simulink model "two_parallel_full_model_simscape"  (R2023b)
settings: Solver=ode1be  StartTime=0.0  StopTime=simlength  FixedStep=ts_sim  MaxStep=ts_sim
undefined symbols (not defined in the file): fclock, fPWM_INV, fPWM_ZVS, gate_nominal_voltage, I_FS, Iout_dc_nom, ki_i_inv, ki_i_zvs, ki_v_inv, ki_v_zvs, kp_i_inv, kp_i_zvs, kp_v_inv, kp_v_zvs, LFi_dc, LFu_ac, magnitude, n10, omega_grid, RCFu_dc, RLFi_dc, RLFu_ac, tc, Tc, tPWM_ZVS, ts_afe, ts_inv, ts_zvs, ugrid_factor, Ugrid_phase_normalization_factor, un_eta_pu, un_xi_pu, up_xi_pu, v1_trafo, v2_trafo, V_FS, Vout_dc_nom
libraries: fl_lib x142, nesl_utility x55, single_phase_transformer_lib x4
(part 4 of 4)

== system two_parallel_full_model_simscape/zvs_modA/dc//dc with galvanic isolation/stage-1/h-bridge ==
  gate_commands : Inport
  Bus Selector : BusSelector  OutputSignals=gate_Q1,gate_Q2,gate_Q3,gate_Q4
  Current Sensor1 : fl_lib/Electrical/Electrical Sensors/Current Sensor
  Simulink-PS Converter{,1..3} (4 alike) : nesl_utility/Simulink-PS Converter  PhysicalDomain=network_engine_domain  SubClassName=ps_input  LeftPortType=input  RightPortType=output  PseudoPeriodic=off  Frequencies=[]  NoiseDistribution=none  NoiseParameters=[]  Unit=1  AffineConversion=on  FilteringAndDerivatives=provide  SimscapeFilterOrder=1  InputFilterTimeConstant=0.001  UdotUserProvided=0
  ileg_dc_inv : nesl_utility/PS-Simulink Converter  PhysicalDomain=network_engine_domain  SubClassName=ps_output  LeftPortType=input  RightPortType=output  PseudoPeriodic=off  Frequencies=[]  VectorFormat=1-D array  Unit=A  AffineConversion=on
  switch_1 : Subsystem
      settings: PortSchema="{\"entries\":[{\"content\":{\"sides\":[{\"content\":{\"connectorIds\":[\"LConn1\"]},\"type\":\"ConnectorPlacement.EquallySpacedRectSide\",\"uuid\":\"9277da8d-d460-43e6-8478-dd662f15d226\"},{\"content\":{\"connectorIds\":[],\"side\":\"RIGHT\"},\"type\":\"ConnectorPlacement.EquallySpacedRectSide\",\"uuid\":\"a7ece396-f1d9-4f4f-a05b-db1fc65d6e1d\"},{\"content\":{\"connectorIds\":[\"LConn2\"],\"side\":\"TOP\"},\"type\":\"ConnectorPlacement.EquallySpacedRectSide\",\"uuid\":\"fdd70777-e9cf-4317-afb6-cae87f75d5b0\"},{\"content\":{\"connectorIds\":[\"RConn1\"],\"side\":\"BOTTOM\"},\"type\":\"ConnectorPlacement.EquallySpacedRectSide\",\"uuid\":\"2353ed68-b1a1-4775-9ca9-31e268d5443b\"}]},\"type\":\"ConnectorPlacement.EquallySpacedConnector\",\"uuid\":\"d5479f4c-4e65-4791-adcb-73df11f88590\"}],\"packageUris\":[\"http://schema.mathworks.com/mf0/Connector/R2020b\"],\"version\":\"1.0\"}"
  switch_2 : Subsystem
      settings: PortSchema="{\"entries\":[{\"content\":{\"sides\":[{\"content\":{\"connectorIds\":[\"LConn1\"]},\"type\":\"ConnectorPlacement.EquallySpacedRectSide\",\"uuid\":\"9277da8d-d460-43e6-8478-dd662f15d226\"},{\"content\":{\"connectorIds\":[],\"side\":\"RIGHT\"},\"type\":\"ConnectorPlacement.EquallySpacedRectSide\",\"uuid\":\"a7ece396-f1d9-4f4f-a05b-db1fc65d6e1d\"},{\"content\":{\"connectorIds\":[\"LConn2\"],\"side\":\"TOP\"},\"type\":\"ConnectorPlacement.EquallySpacedRectSide\",\"uuid\":\"fdd70777-e9cf-4317-afb6-cae87f75d5b0\"},{\"content\":{\"connectorIds\":[\"RConn1\"],\"side\":\"BOTTOM\"},\"type\":\"ConnectorPlacement.EquallySpacedRectSide\",\"uuid\":\"2353ed68-b1a1-4775-9ca9-31e268d5443b\"}]},\"type\":\"ConnectorPlacement.EquallySpacedConnector\",\"uuid\":\"d5479f4c-4e65-4791-adcb-73df11f88590\"}],\"packageUris\":[\"http://schema.mathworks.com/mf0/Connector/R2020b\"],\"version\":\"1.0\"}"
  switch_3 : Subsystem
      settings: PortSchema="{\"entries\":[{\"content\":{\"sides\":[{\"content\":{\"connectorIds\":[\"LConn1\"]},\"type\":\"ConnectorPlacement.EquallySpacedRectSide\",\"uuid\":\"9277da8d-d460-43e6-8478-dd662f15d226\"},{\"content\":{\"connectorIds\":[],\"side\":\"RIGHT\"},\"type\":\"ConnectorPlacement.EquallySpacedRectSide\",\"uuid\":\"a7ece396-f1d9-4f4f-a05b-db1fc65d6e1d\"},{\"content\":{\"connectorIds\":[\"LConn2\"],\"side\":\"TOP\"},\"type\":\"ConnectorPlacement.EquallySpacedRectSide\",\"uuid\":\"fdd70777-e9cf-4317-afb6-cae87f75d5b0\"},{\"content\":{\"connectorIds\":[\"RConn1\"],\"side\":\"BOTTOM\"},\"type\":\"ConnectorPlacement.EquallySpacedRectSide\",\"uuid\":\"2353ed68-b1a1-4775-9ca9-31e268d5443b\"}]},\"type\":\"ConnectorPlacement.EquallySpacedConnector\",\"uuid\":\"d5479f4c-4e65-4791-adcb-73df11f88590\"}],\"packageUris\":[\"http://schema.mathworks.com/mf0/Connector/R2020b\"],\"version\":\"1.0\"}"
  switch_4 : Subsystem
      settings: PortSchema="{\"entries\":[{\"content\":{\"sides\":[{\"content\":{\"connectorIds\":[\"LConn1\"]},\"type\":\"ConnectorPlacement.EquallySpacedRectSide\",\"uuid\":\"9277da8d-d460-43e6-8478-dd662f15d226\"},{\"content\":{\"connectorIds\":[],\"side\":\"RIGHT\"},\"type\":\"ConnectorPlacement.EquallySpacedRectSide\",\"uuid\":\"a7ece396-f1d9-4f4f-a05b-db1fc65d6e1d\"},{\"content\":{\"connectorIds\":[\"LConn2\"],\"side\":\"TOP\"},\"type\":\"ConnectorPlacement.EquallySpacedRectSide\",\"uuid\":\"fdd70777-e9cf-4317-afb6-cae87f75d5b0\"},{\"content\":{\"connectorIds\":[\"RConn1\"],\"side\":\"BOTTOM\"},\"type\":\"ConnectorPlacement.EquallySpacedRectSide\",\"uuid\":\"2353ed68-b1a1-4775-9ca9-31e268d5443b\"}]},\"type\":\"ConnectorPlacement.EquallySpacedConnector\",\"uuid\":\"d5479f4c-4e65-4791-adcb-73df11f88590\"}],\"packageUris\":[\"http://schema.mathworks.com/mf0/Connector/R2020b\"],\"version\":\"1.0\"}"
  uac_1(+) : PMIOPort  Side=Left
  uac_1(-) : PMIOPort  Port=2  Side=Left
  udc(+) : PMIOPort  Port=3  Side=Right
  udc(-) : PMIOPort  Port=4  Side=Right
  tag scope: ileg_dc_inv=global
  wires:
  [gate_Q1] -> Simulink-PS Converter/1
  [gate_Q2] -> Simulink-PS Converter1/1
  [gate_Q3] -> Simulink-PS Converter2/1
  [gate_Q4] -> Simulink-PS Converter3/1
  gate_commands/1 -> Bus Selector/1
  ileg_dc_inv/1 -> [ileg_dc_inv]
  Bus Selector/1 -> [gate_Q1]  "<gate_Q1>"
  Bus Selector/2 -> [gate_Q2]  "<gate_Q2>"
  Bus Selector/3 -> [gate_Q3]  "<gate_Q3>"
  Bus Selector/4 -> [gate_Q4]  "<gate_Q4>"
  connections:
  Current Sensor1/LConn1 -- switch_3/LConn2 -- udc(+)/RConn1
  udc(-)/RConn1 -- switch_4/RConn1 -- switch_2/RConn1
  Simulink-PS Converter/RConn1 -- switch_1/LConn1
  switch_2/LConn1 -- Simulink-PS Converter1/RConn1
  switch_3/LConn1 -- Simulink-PS Converter2/RConn1
  switch_4/LConn1 -- Simulink-PS Converter3/RConn1
  uac_1(+)/RConn1 -- switch_2/LConn2 -- switch_1/RConn1
  uac_1(-)/RConn1 -- switch_4/LConn2 -- switch_3/RConn1
  Current Sensor1/RConn2 -- switch_1/LConn2
  Current Sensor1/RConn1 -- ileg_dc_inv/LConn1

== system two_parallel_full_model_simscape/zvs_modA/dc//dc with galvanic isolation/stage-2/two-phase-rectifier_tr1 ==
  Diode{,1,3..4} (4 alike) : fl_lib/Electrical/Electrical Elements/Diode  Vf=Vdon_diode V  Ron=Rdon_diode Ohm  Goff=1e-8 1/Ohm  i_specify=off  i_priority=None  i=0 A  i_nominal_specify=off  i_nominal_unit=A  i_nominal_value=1  v_specify=off  v_priority=None  v=0 V  v_nominal_specify=off  v_nominal_unit=V  v_nominal_value=1
  udc(+) : PMIOPort  Side=Right
  uac(+) : PMIOPort  Port=2  Side=Left
  uac(-) : PMIOPort  Port=3  Side=Left
  udc(-) : PMIOPort  Port=4  Side=Right
  connections:
  Diode/LConn1 -- Diode3/RConn1 -- uac(+)/RConn1
  Diode/RConn1 -- udc(+)/RConn1 -- Diode1/RConn1
  Diode3/LConn1 -- udc(-)/RConn1 -- Diode4/LConn1
  Diode4/RConn1 -- Diode1/LConn1 -- uac(-)/RConn1

== system two_parallel_full_model_simscape/zvs_modA/dc//dc with galvanic isolation/stage-2/two-phase-rectifier_tr2 ==
  Diode{,1,3..4} (4 alike) : fl_lib/Electrical/Electrical Elements/Diode  Vf=Vdon_diode V  Ron=Rdon_diode Ohm  Goff=1e-8 1/Ohm  i_specify=off  i_priority=None  i=0 A  i_nominal_specify=off  i_nominal_unit=A  i_nominal_value=1  v_specify=off  v_priority=None  v=0 V  v_nominal_specify=off  v_nominal_unit=V  v_nominal_value=1
  udc(+) : PMIOPort  Side=Right
  uac(+) : PMIOPort  Port=2  Side=Left
  uac(-) : PMIOPort  Port=3  Side=Left
  udc(-) : PMIOPort  Port=4  Side=Right
  connections:
  uac(-)/RConn1 -- Diode4/RConn1 -- Diode1/LConn1
  udc(-)/RConn1 -- Diode4/LConn1 -- Diode3/LConn1
  udc(+)/RConn1 -- Diode1/RConn1 -- Diode/RConn1
  uac(+)/RConn1 -- Diode3/RConn1 -- Diode/LConn1

== system two_parallel_full_model_simscape/zvs_modA/zvs_ctrl/references/voltage_reference ==
  Constant1 : Constant  Value=Vout_dc_nom
  Manual Switch : ManualSwitch
  Rate Limiter : RateLimiter  RisingSlewLimit=Vout_dc_nom  FallingSlewLimit=-Vout_dc_nom  SampleTimeMode=inherited
  Step : Step  Time=0.25  After=20  SampleTime=0
  Step1 : Step  Time=0.45  After=480  SampleTime=0
  Step2 : Step  Time=0.75  After=480  SampleTime=0
  Step3 : Step  After=780  SampleTime=0
  Sum : Sum  Inputs=|++
  Sum1 : Sum  Inputs=|+-
  Sum2 : Sum  Inputs=|++
  To Workspace2 : ToWorkspace  VariableName=vout_ref_modA_sim  SampleTime=ts_zvs
      settings: MaxDataPoints=Ns_zvs
  Vout_dc_nom : Step  Time=1e-3  After=Vout_dc_nom  SampleTime=0
  vout_ref : Outport
  wires:
  Step/1 -> Sum/1
  Step1/1 -> Sum/2
  Sum/1 -> Sum1/1
  Step2/1 -> Sum1/2
  Sum1/1 -> Sum2/1
  Step3/1 -> Sum2/2
  Sum2/1 -> Manual Switch/2
  Vout_dc_nom/1 -> Rate Limiter/1
  Manual Switch/1 -> To Workspace2/1, vout_ref/1
  Rate Limiter/1 -> Manual Switch/1

== system two_parallel_full_model_simscape/zvs_modA/zvs_ctrl/vi ctrl/Iout Ctrl ==
  iout_ref : Inport
  iout : Inport  Port=2
  Product : Product
  Rate Limiter : RateLimiter  FallingSlewLimit=0  SampleTimeMode=inherited
  Saturation1 : Saturate  UpperLimit=1  LowerLimit=0  OutDataTypeStr=double
  Step : Step  Time=0.1  SampleTime=0
  Sum2 : Sum  Inputs=+-  OutDataTypeStr=double  AccumDataTypeStr=double  SaturateOnIntegerOverflow=on
  To Workspace2 : ToWorkspace  VariableName=iout_ref_dsp_modA_sim  SampleTime=ts_zvs
      settings: MaxDataPoints=Ns_zvs
  To Workspace9 : ToWorkspace  VariableName=iout_dsp_modA_sim  SampleTime=ts_zvs
      settings: MaxDataPoints=Ns_zvs
  iout_ctrl : Subsystem
  ctrli_out : Outport
  wires:
  iout_ctrl/1(ctrli_out) -> ctrli_out/1
  iout/1 -> To Workspace9/1, Sum2/2
  iout_ref/1 -> Sum2/1, To Workspace2/1
  Rate Limiter/1 -> Saturation1/1
  Saturation1/1 -> Product/1
  Step/1 -> Rate Limiter/1
  Sum2/1 -> Product/2
  Product/1 -> iout_ctrl/1(i_tilde)

== system two_parallel_full_model_simscape/zvs_modA/zvs_ctrl/vi ctrl/Vout Ctrl ==
  vout_ref : Inport
  vout : Inport  Port=2
  Product : Product
  Rate Limiter : RateLimiter  FallingSlewLimit=0  SampleTimeMode=inherited
  Saturation1 : Saturate  UpperLimit=1  LowerLimit=0  OutDataTypeStr=double
  Step : Step  Time=0.1  SampleTime=0
  Sum2 : Sum  Inputs=+-  OutDataTypeStr=double  AccumDataTypeStr=double  SaturateOnIntegerOverflow=on
  To Workspace2 : ToWorkspace  VariableName=vout_ref_dsp_modA_sim  SampleTime=ts_zvs
      settings: MaxDataPoints=Ns_zvs
  To Workspace9 : ToWorkspace  VariableName=vout_dsp_modA_sim  SampleTime=ts_zvs
      settings: MaxDataPoints=Ns_zvs
  vout_ctrl : Subsystem
  ctrlv_out : Outport
  wires:
  vout_ref/1 -> To Workspace2/1, Sum2/1
  vout/1 -> To Workspace9/1, Sum2/2
  vout_ctrl/1(ctrlv_out) -> ctrlv_out/1
  Sum2/1 -> Product/2
  Product/1 -> vout_ctrl/1(ixi_tilde)
  Step/1 -> Rate Limiter/1
  Rate Limiter/1 -> Saturation1/1
  Saturation1/1 -> Product/1

== system two_parallel_full_model_simscape/zvs_modB/dc//dc with galvanic isolation/stage-1/h-bridge ==
  gate_commands : Inport
  Bus Selector : BusSelector  OutputSignals=gate_Q1,gate_Q2,gate_Q3,gate_Q4
  Simulink-PS Converter{,1..3} (4 alike) : nesl_utility/Simulink-PS Converter  PhysicalDomain=network_engine_domain  SubClassName=ps_input  LeftPortType=input  RightPortType=output  PseudoPeriodic=off  Frequencies=[]  NoiseDistribution=none  NoiseParameters=[]  Unit=1  AffineConversion=on  FilteringAndDerivatives=provide  SimscapeFilterOrder=1  InputFilterTimeConstant=0.001  UdotUserProvided=0
  switch_1 : Subsystem
      settings: PortSchema="{\"entries\":[{\"content\":{\"sides\":[{\"content\":{\"connectorIds\":[\"LConn1\"]},\"type\":\"ConnectorPlacement.EquallySpacedRectSide\",\"uuid\":\"9277da8d-d460-43e6-8478-dd662f15d226\"},{\"content\":{\"connectorIds\":[],\"side\":\"RIGHT\"},\"type\":\"ConnectorPlacement.EquallySpacedRectSide\",\"uuid\":\"a7ece396-f1d9-4f4f-a05b-db1fc65d6e1d\"},{\"content\":{\"connectorIds\":[\"LConn2\"],\"side\":\"TOP\"},\"type\":\"ConnectorPlacement.EquallySpacedRectSide\",\"uuid\":\"fdd70777-e9cf-4317-afb6-cae87f75d5b0\"},{\"content\":{\"connectorIds\":[\"RConn1\"],\"side\":\"BOTTOM\"},\"type\":\"ConnectorPlacement.EquallySpacedRectSide\",\"uuid\":\"2353ed68-b1a1-4775-9ca9-31e268d5443b\"}]},\"type\":\"ConnectorPlacement.EquallySpacedConnector\",\"uuid\":\"d5479f4c-4e65-4791-adcb-73df11f88590\"}],\"packageUris\":[\"http://schema.mathworks.com/mf0/Connector/R2020b\"],\"version\":\"1.0\"}"
  switch_2 : Subsystem
      settings: PortSchema="{\"entries\":[{\"content\":{\"sides\":[{\"content\":{\"connectorIds\":[\"LConn1\"]},\"type\":\"ConnectorPlacement.EquallySpacedRectSide\",\"uuid\":\"9277da8d-d460-43e6-8478-dd662f15d226\"},{\"content\":{\"connectorIds\":[],\"side\":\"RIGHT\"},\"type\":\"ConnectorPlacement.EquallySpacedRectSide\",\"uuid\":\"a7ece396-f1d9-4f4f-a05b-db1fc65d6e1d\"},{\"content\":{\"connectorIds\":[\"LConn2\"],\"side\":\"TOP\"},\"type\":\"ConnectorPlacement.EquallySpacedRectSide\",\"uuid\":\"fdd70777-e9cf-4317-afb6-cae87f75d5b0\"},{\"content\":{\"connectorIds\":[\"RConn1\"],\"side\":\"BOTTOM\"},\"type\":\"ConnectorPlacement.EquallySpacedRectSide\",\"uuid\":\"2353ed68-b1a1-4775-9ca9-31e268d5443b\"}]},\"type\":\"ConnectorPlacement.EquallySpacedConnector\",\"uuid\":\"d5479f4c-4e65-4791-adcb-73df11f88590\"}],\"packageUris\":[\"http://schema.mathworks.com/mf0/Connector/R2020b\"],\"version\":\"1.0\"}"
  switch_3 : Subsystem
      settings: PortSchema="{\"entries\":[{\"content\":{\"sides\":[{\"content\":{\"connectorIds\":[\"LConn1\"]},\"type\":\"ConnectorPlacement.EquallySpacedRectSide\",\"uuid\":\"9277da8d-d460-43e6-8478-dd662f15d226\"},{\"content\":{\"connectorIds\":[],\"side\":\"RIGHT\"},\"type\":\"ConnectorPlacement.EquallySpacedRectSide\",\"uuid\":\"a7ece396-f1d9-4f4f-a05b-db1fc65d6e1d\"},{\"content\":{\"connectorIds\":[\"LConn2\"],\"side\":\"TOP\"},\"type\":\"ConnectorPlacement.EquallySpacedRectSide\",\"uuid\":\"fdd70777-e9cf-4317-afb6-cae87f75d5b0\"},{\"content\":{\"connectorIds\":[\"RConn1\"],\"side\":\"BOTTOM\"},\"type\":\"ConnectorPlacement.EquallySpacedRectSide\",\"uuid\":\"2353ed68-b1a1-4775-9ca9-31e268d5443b\"}]},\"type\":\"ConnectorPlacement.EquallySpacedConnector\",\"uuid\":\"d5479f4c-4e65-4791-adcb-73df11f88590\"}],\"packageUris\":[\"http://schema.mathworks.com/mf0/Connector/R2020b\"],\"version\":\"1.0\"}"
  switch_4 : Subsystem
      settings: PortSchema="{\"entries\":[{\"content\":{\"sides\":[{\"content\":{\"connectorIds\":[\"LConn1\"]},\"type\":\"ConnectorPlacement.EquallySpacedRectSide\",\"uuid\":\"9277da8d-d460-43e6-8478-dd662f15d226\"},{\"content\":{\"connectorIds\":[],\"side\":\"RIGHT\"},\"type\":\"ConnectorPlacement.EquallySpacedRectSide\",\"uuid\":\"a7ece396-f1d9-4f4f-a05b-db1fc65d6e1d\"},{\"content\":{\"connectorIds\":[\"LConn2\"],\"side\":\"TOP\"},\"type\":\"ConnectorPlacement.EquallySpacedRectSide\",\"uuid\":\"fdd70777-e9cf-4317-afb6-cae87f75d5b0\"},{\"content\":{\"connectorIds\":[\"RConn1\"],\"side\":\"BOTTOM\"},\"type\":\"ConnectorPlacement.EquallySpacedRectSide\",\"uuid\":\"2353ed68-b1a1-4775-9ca9-31e268d5443b\"}]},\"type\":\"ConnectorPlacement.EquallySpacedConnector\",\"uuid\":\"d5479f4c-4e65-4791-adcb-73df11f88590\"}],\"packageUris\":[\"http://schema.mathworks.com/mf0/Connector/R2020b\"],\"version\":\"1.0\"}"
  uac_1(+) : PMIOPort  Side=Left
  uac_1(-) : PMIOPort  Port=2  Side=Left
  udc(+) : PMIOPort  Port=3  Side=Right
  udc(-) : PMIOPort  Port=4  Side=Right
  wires:
  Bus Selector/4 -> [gate_Q4]  "<gate_Q4>"
  Bus Selector/3 -> [gate_Q3]  "<gate_Q3>"
  Bus Selector/2 -> [gate_Q2]  "<gate_Q2>"
  Bus Selector/1 -> [gate_Q1]  "<gate_Q1>"
  gate_commands/1 -> Bus Selector/1
  [gate_Q4] -> Simulink-PS Converter3/1
  [gate_Q3] -> Simulink-PS Converter2/1
  [gate_Q2] -> Simulink-PS Converter1/1
  [gate_Q1] -> Simulink-PS Converter/1
  connections:
  switch_3/RConn1 -- switch_4/LConn2 -- uac_1(-)/RConn1
  switch_1/RConn1 -- switch_2/LConn2 -- uac_1(+)/RConn1
  switch_4/LConn1 -- Simulink-PS Converter3/RConn1
  switch_3/LConn1 -- Simulink-PS Converter2/RConn1
  switch_2/LConn1 -- Simulink-PS Converter1/RConn1
  Simulink-PS Converter/RConn1 -- switch_1/LConn1
  switch_2/RConn1 -- switch_4/RConn1 -- udc(-)/RConn1
  udc(+)/RConn1 -- switch_3/LConn2 -- switch_1/LConn2

== system two_parallel_full_model_simscape/zvs_modB/dc//dc with galvanic isolation/stage-2/two-phase-rectifier_tr1 ==
  Diode{,1,3..4} (4 alike) : fl_lib/Electrical/Electrical Elements/Diode  Vf=Vdon_diode V  Ron=Rdon_diode Ohm  Goff=1e-8 1/Ohm  i_specify=off  i_priority=None  i=0 A  i_nominal_specify=off  i_nominal_unit=A  i_nominal_value=1  v_specify=off  v_priority=None  v=0 V  v_nominal_specify=off  v_nominal_unit=V  v_nominal_value=1
  udc(+) : PMIOPort  Side=Right
  uac(+) : PMIOPort  Port=2  Side=Left
  uac(-) : PMIOPort  Port=3  Side=Left
  udc(-) : PMIOPort  Port=4  Side=Right
  connections:
  uac(-)/RConn1 -- Diode1/LConn1 -- Diode4/RConn1
  Diode4/LConn1 -- udc(-)/RConn1 -- Diode3/LConn1
  Diode1/RConn1 -- udc(+)/RConn1 -- Diode/RConn1
  uac(+)/RConn1 -- Diode3/RConn1 -- Diode/LConn1

== system two_parallel_full_model_simscape/zvs_modB/dc//dc with galvanic isolation/stage-2/two-phase-rectifier_tr2 ==
  Diode{,1,3..4} (4 alike) : fl_lib/Electrical/Electrical Elements/Diode  Vf=Vdon_diode V  Ron=Rdon_diode Ohm  Goff=1e-8 1/Ohm  i_specify=off  i_priority=None  i=0 A  i_nominal_specify=off  i_nominal_unit=A  i_nominal_value=1  v_specify=off  v_priority=None  v=0 V  v_nominal_specify=off  v_nominal_unit=V  v_nominal_value=1
  udc(+) : PMIOPort  Side=Right
  uac(+) : PMIOPort  Port=2  Side=Left
  uac(-) : PMIOPort  Port=3  Side=Left
  udc(-) : PMIOPort  Port=4  Side=Right
  connections:
  Diode/LConn1 -- Diode3/RConn1 -- uac(+)/RConn1
  Diode/RConn1 -- Diode1/RConn1 -- udc(+)/RConn1
  Diode3/LConn1 -- Diode4/LConn1 -- udc(-)/RConn1
  Diode1/LConn1 -- Diode4/RConn1 -- uac(-)/RConn1

== system two_parallel_full_model_simscape/zvs_modB/zvs_ctrl/references/voltage_reference ==
  Constant1 : Constant  Value=Vout_dc_nom
  Manual Switch : ManualSwitch
  Rate Limiter : RateLimiter  RisingSlewLimit=Vout_dc_nom  FallingSlewLimit=-Vout_dc_nom  SampleTimeMode=inherited
  Step : Step  Time=0.25  After=20  SampleTime=0
  Step1 : Step  Time=0.45  After=480  SampleTime=0
  Step2 : Step  Time=0.75  After=480  SampleTime=0
  Step3 : Step  After=780  SampleTime=0
  Sum : Sum  Inputs=|++
  Sum1 : Sum  Inputs=|+-
  Sum2 : Sum  Inputs=|++
  Vout_dc_nom : Step  Time=1e-3  After=Vout_dc_nom  SampleTime=0
  vout_ref : Outport
  wires:
  Rate Limiter/1 -> Manual Switch/1
  Manual Switch/1 -> vout_ref/1
  Vout_dc_nom/1 -> Rate Limiter/1
  Sum2/1 -> Manual Switch/2
  Step3/1 -> Sum2/2
  Sum1/1 -> Sum2/1
  Step2/1 -> Sum1/2
  Sum/1 -> Sum1/1
  Step1/1 -> Sum/2
  Step/1 -> Sum/1

== system two_parallel_full_model_simscape/zvs_modB/zvs_ctrl/vi ctrl/Iout Ctrl ==
  iout_ref : Inport
  iout : Inport  Port=2
  Product : Product
  Rate Limiter : RateLimiter  FallingSlewLimit=0  SampleTimeMode=inherited
  Saturation1 : Saturate  UpperLimit=1  LowerLimit=0  OutDataTypeStr=double
  Step : Step  Time=0.1  SampleTime=0
  Sum2 : Sum  Inputs=+-  OutDataTypeStr=double  AccumDataTypeStr=double  SaturateOnIntegerOverflow=on
  To Workspace2 : ToWorkspace  VariableName=iout_ref_dsp_modB_sim  SampleTime=ts_zvs
      settings: MaxDataPoints=Ns_zvs
  To Workspace9 : ToWorkspace  VariableName=iout_dsp_modB_sim  SampleTime=ts_zvs
      settings: MaxDataPoints=Ns_zvs
  iout_ctrl : Subsystem
  ctrli_out : Outport
  wires:
  Product/1 -> iout_ctrl/1(i_tilde)
  Sum2/1 -> Product/2
  Step/1 -> Rate Limiter/1
  Saturation1/1 -> Product/1
  Rate Limiter/1 -> Saturation1/1
  iout_ref/1 -> To Workspace2/1, Sum2/1
  iout/1 -> Sum2/2, To Workspace9/1
  iout_ctrl/1(ctrli_out) -> ctrli_out/1

== system two_parallel_full_model_simscape/zvs_modB/zvs_ctrl/vi ctrl/Vout Ctrl ==
  vout_ref : Inport
  vout : Inport  Port=2
  Product : Product
  Rate Limiter : RateLimiter  FallingSlewLimit=0  SampleTimeMode=inherited
  Saturation1 : Saturate  UpperLimit=1  LowerLimit=0  OutDataTypeStr=double
  Step : Step  Time=0.1  SampleTime=0
  Sum2 : Sum  Inputs=+-  OutDataTypeStr=double  AccumDataTypeStr=double  SaturateOnIntegerOverflow=on
  To Workspace2 : ToWorkspace  VariableName=vout_ref_dsp_modB_sim  SampleTime=ts_zvs
      settings: MaxDataPoints=Ns_zvs
  To Workspace9 : ToWorkspace  VariableName=vout_dsp_modB_sim  SampleTime=ts_zvs
      settings: MaxDataPoints=Ns_zvs
  vout_ctrl : Subsystem
  ctrlv_out : Outport
  wires:
  Saturation1/1 -> Product/1
  Rate Limiter/1 -> Saturation1/1
  Step/1 -> Rate Limiter/1
  Product/1 -> vout_ctrl/1(ixi_tilde)
  Sum2/1 -> Product/2
  vout_ctrl/1(ctrlv_out) -> ctrlv_out/1
  vout/1 -> Sum2/2, To Workspace9/1
  vout_ref/1 -> Sum2/1, To Workspace2/1

== system two_parallel_full_model_simscape/zvs_modA/dc//dc with galvanic isolation/stage-1/h-bridge/switch_1 ==
  Diode : fl_lib/Electrical/Electrical Elements/Diode  Vf=Vdon_diode V  Ron=Rdon_diode Ohm  Goff=1e-8 1/Ohm  i_specify=off  i_priority=None  i=0 A  i_nominal_specify=off  i_nominal_unit=A  i_nominal_value=1  v_specify=off  v_priority=None  v=0 V  v_nominal_specify=off  v_nominal_unit=V  v_nominal_value=1
  Switch : fl_lib/Electrical/Electrical Elements/Switch  R_closed=Ron Ohm  G_open=1e-8 1/Ohm  Threshold=7.5  i_specify=off  i_priority=None  i=0 A  i_nominal_specify=off  i_nominal_unit=A  i_nominal_value=1  v_specify=off  v_priority=None  v=0 V  v_nominal_specify=off  v_nominal_unit=V  v_nominal_value=1
  G : PMIOPort  Side=Left
  C : PMIOPort  Port=2  Side=Left
  E : PMIOPort  Port=3  Side=Right
  connections:
  Switch/RConn2 -- C/RConn1 -- Diode/RConn1
  Switch/RConn1 -- G/RConn1
  Switch/LConn1 -- E/RConn1 -- Diode/LConn1

== system two_parallel_full_model_simscape/zvs_modA/dc//dc with galvanic isolation/stage-1/h-bridge/switch_2 ==
  Diode : fl_lib/Electrical/Electrical Elements/Diode  Vf=Vdon_diode V  Ron=Rdon_diode Ohm  Goff=1e-8 1/Ohm  i_specify=off  i_priority=None  i=0 A  i_nominal_specify=off  i_nominal_unit=A  i_nominal_value=1  v_specify=off  v_priority=None  v=0 V  v_nominal_specify=off  v_nominal_unit=V  v_nominal_value=1
  Switch : fl_lib/Electrical/Electrical Elements/Switch  R_closed=Ron Ohm  G_open=1e-8 1/Ohm  Threshold=7.5  i_specify=off  i_priority=None  i=0 A  i_nominal_specify=off  i_nominal_unit=A  i_nominal_value=1  v_specify=off  v_priority=None  v=0 V  v_nominal_specify=off  v_nominal_unit=V  v_nominal_value=1
  G : PMIOPort  Side=Left
  C : PMIOPort  Port=2  Side=Left
  E : PMIOPort  Port=3  Side=Right
  connections:
  Diode/LConn1 -- E/RConn1 -- Switch/LConn1
  Switch/RConn1 -- G/RConn1
  Diode/RConn1 -- C/RConn1 -- Switch/RConn2

== system two_parallel_full_model_simscape/zvs_modA/dc//dc with galvanic isolation/stage-1/h-bridge/switch_3 ==
  Diode : fl_lib/Electrical/Electrical Elements/Diode  Vf=Vdon_diode V  Ron=Rdon_diode Ohm  Goff=1e-8 1/Ohm  i_specify=off  i_priority=None  i=0 A  i_nominal_specify=off  i_nominal_unit=A  i_nominal_value=1  v_specify=off  v_priority=None  v=0 V  v_nominal_specify=off  v_nominal_unit=V  v_nominal_value=1
  Switch : fl_lib/Electrical/Electrical Elements/Switch  R_closed=Ron Ohm  G_open=1e-8 1/Ohm  Threshold=7.5  i_specify=off  i_priority=None  i=0 A  i_nominal_specify=off  i_nominal_unit=A  i_nominal_value=1  v_specify=off  v_priority=None  v=0 V  v_nominal_specify=off  v_nominal_unit=V  v_nominal_value=1
  G : PMIOPort  Side=Left
  C : PMIOPort  Port=2  Side=Left
  E : PMIOPort  Port=3  Side=Right
  connections:
  Switch/RConn2 -- C/RConn1 -- Diode/RConn1
  Switch/RConn1 -- G/RConn1
  Switch/LConn1 -- E/RConn1 -- Diode/LConn1

== system two_parallel_full_model_simscape/zvs_modA/dc//dc with galvanic isolation/stage-1/h-bridge/switch_4 ==
  Diode : fl_lib/Electrical/Electrical Elements/Diode  Vf=Vdon_diode V  Ron=Rdon_diode Ohm  Goff=1e-8 1/Ohm  i_specify=off  i_priority=None  i=0 A  i_nominal_specify=off  i_nominal_unit=A  i_nominal_value=1  v_specify=off  v_priority=None  v=0 V  v_nominal_specify=off  v_nominal_unit=V  v_nominal_value=1
  Switch : fl_lib/Electrical/Electrical Elements/Switch  R_closed=Ron Ohm  G_open=1e-8 1/Ohm  Threshold=7.5  i_specify=off  i_priority=None  i=0 A  i_nominal_specify=off  i_nominal_unit=A  i_nominal_value=1  v_specify=off  v_priority=None  v=0 V  v_nominal_specify=off  v_nominal_unit=V  v_nominal_value=1
  G : PMIOPort  Side=Left
  C : PMIOPort  Port=2  Side=Left
  E : PMIOPort  Port=3  Side=Right
  connections:
  Diode/LConn1 -- E/RConn1 -- Switch/LConn1
  Switch/RConn1 -- G/RConn1
  Diode/RConn1 -- C/RConn1 -- Switch/RConn2

== system two_parallel_full_model_simscape/zvs_modA/zvs_ctrl/vi ctrl/Iout Ctrl/iout_ctrl ==
  i_tilde : Inport
  1/Ti : Gain  Gain=kp_i_zvs  ParamDataTypeStr=double  OutDataTypeStr=double  SaturateOnIntegerOverflow=on
  Saturation2 : Saturate  UpperLimit=1  LowerLimit=0  OutDataTypeStr=double
  Sum1 : Sum  Inputs=+++  SaturateOnIntegerOverflow=on
  Sum4 : Sum  Inputs=-+  SaturateOnIntegerOverflow=on
  Unit Delay4 : UnitDelay  SampleTime=ts_zvs  HasFrameUpgradeWarning=on
  kp2 : Gain  Gain=ki_i_zvs*ts_zvs  ParamDataTypeStr=double  OutDataTypeStr=double  SaturateOnIntegerOverflow=on
  ctrli_out : Outport
  wires:
  i_tilde/1 -> kp2/1, 1/Ti/1
  Sum1/1 -> Saturation2/1
  Saturation2/1 -> Sum4/2, ctrli_out/1
  kp2/1 -> Sum1/2
  1/Ti/1 -> Sum1/1, Sum4/1
  Sum4/1 -> Unit Delay4/1
  Unit Delay4/1 -> Sum1/3

== system two_parallel_full_model_simscape/zvs_modA/zvs_ctrl/vi ctrl/Vout Ctrl/vout_ctrl ==
  ixi_tilde : Inport
  1/Ti : Gain  Gain=kp_v_zvs  ParamDataTypeStr=double  OutDataTypeStr=double  SaturateOnIntegerOverflow=on
  Saturation2 : Saturate  UpperLimit=1  LowerLimit=0  OutDataTypeStr=double
  Sum1 : Sum  Inputs=+++  SaturateOnIntegerOverflow=on
  Sum4 : Sum  Inputs=-+  SaturateOnIntegerOverflow=on
  Unit Delay4 : UnitDelay  SampleTime=ts_zvs  HasFrameUpgradeWarning=on
  kp2 : Gain  Gain=ki_v_zvs*ts_zvs  ParamDataTypeStr=double  OutDataTypeStr=double  SaturateOnIntegerOverflow=on
  ctrlv_out : Outport
  wires:
  ixi_tilde/1 -> kp2/1, 1/Ti/1
  kp2/1 -> Sum1/2
  Sum4/1 -> Unit Delay4/1
  1/Ti/1 -> Sum1/1, Sum4/1
  Sum1/1 -> Saturation2/1
  Unit Delay4/1 -> Sum1/3
  Saturation2/1 -> ctrlv_out/1, Sum4/2

== system two_parallel_full_model_simscape/zvs_modB/dc//dc with galvanic isolation/stage-1/h-bridge/switch_1 ==
  Diode : fl_lib/Electrical/Electrical Elements/Diode  Vf=Vdon_diode V  Ron=Rdon_diode Ohm  Goff=1e-8 1/Ohm  i_specify=off  i_priority=None  i=0 A  i_nominal_specify=off  i_nominal_unit=A  i_nominal_value=1  v_specify=off  v_priority=None  v=0 V  v_nominal_specify=off  v_nominal_unit=V  v_nominal_value=1
  Switch : fl_lib/Electrical/Electrical Elements/Switch  R_closed=Ron Ohm  G_open=1e-8 1/Ohm  Threshold=7.5  i_specify=off  i_priority=None  i=0 A  i_nominal_specify=off  i_nominal_unit=A  i_nominal_value=1  v_specify=off  v_priority=None  v=0 V  v_nominal_specify=off  v_nominal_unit=V  v_nominal_value=1
  G : PMIOPort  Side=Left
  C : PMIOPort  Port=2  Side=Left
  E : PMIOPort  Port=3  Side=Right
  connections:
  Diode/LConn1 -- E/RConn1 -- Switch/LConn1
  Switch/RConn1 -- G/RConn1
  Diode/RConn1 -- C/RConn1 -- Switch/RConn2

== system two_parallel_full_model_simscape/zvs_modB/dc//dc with galvanic isolation/stage-1/h-bridge/switch_2 ==
  Diode : fl_lib/Electrical/Electrical Elements/Diode  Vf=Vdon_diode V  Ron=Rdon_diode Ohm  Goff=1e-8 1/Ohm  i_specify=off  i_priority=None  i=0 A  i_nominal_specify=off  i_nominal_unit=A  i_nominal_value=1  v_specify=off  v_priority=None  v=0 V  v_nominal_specify=off  v_nominal_unit=V  v_nominal_value=1
  Switch : fl_lib/Electrical/Electrical Elements/Switch  R_closed=Ron Ohm  G_open=1e-8 1/Ohm  Threshold=7.5  i_specify=off  i_priority=None  i=0 A  i_nominal_specify=off  i_nominal_unit=A  i_nominal_value=1  v_specify=off  v_priority=None  v=0 V  v_nominal_specify=off  v_nominal_unit=V  v_nominal_value=1
  G : PMIOPort  Side=Left
  C : PMIOPort  Port=2  Side=Left
  E : PMIOPort  Port=3  Side=Right
  connections:
  Switch/RConn2 -- C/RConn1 -- Diode/RConn1
  Switch/RConn1 -- G/RConn1
  Switch/LConn1 -- E/RConn1 -- Diode/LConn1

== system two_parallel_full_model_simscape/zvs_modB/dc//dc with galvanic isolation/stage-1/h-bridge/switch_3 ==
  Diode : fl_lib/Electrical/Electrical Elements/Diode  Vf=Vdon_diode V  Ron=Rdon_diode Ohm  Goff=1e-8 1/Ohm  i_specify=off  i_priority=None  i=0 A  i_nominal_specify=off  i_nominal_unit=A  i_nominal_value=1  v_specify=off  v_priority=None  v=0 V  v_nominal_specify=off  v_nominal_unit=V  v_nominal_value=1
  Switch : fl_lib/Electrical/Electrical Elements/Switch  R_closed=Ron Ohm  G_open=1e-8 1/Ohm  Threshold=7.5  i_specify=off  i_priority=None  i=0 A  i_nominal_specify=off  i_nominal_unit=A  i_nominal_value=1  v_specify=off  v_priority=None  v=0 V  v_nominal_specify=off  v_nominal_unit=V  v_nominal_value=1
  G : PMIOPort  Side=Left
  C : PMIOPort  Port=2  Side=Left
  E : PMIOPort  Port=3  Side=Right
  connections:
  Diode/LConn1 -- E/RConn1 -- Switch/LConn1
  Switch/RConn1 -- G/RConn1
  Diode/RConn1 -- C/RConn1 -- Switch/RConn2

== system two_parallel_full_model_simscape/zvs_modB/dc//dc with galvanic isolation/stage-1/h-bridge/switch_4 ==
  Diode : fl_lib/Electrical/Electrical Elements/Diode  Vf=Vdon_diode V  Ron=Rdon_diode Ohm  Goff=1e-8 1/Ohm  i_specify=off  i_priority=None  i=0 A  i_nominal_specify=off  i_nominal_unit=A  i_nominal_value=1  v_specify=off  v_priority=None  v=0 V  v_nominal_specify=off  v_nominal_unit=V  v_nominal_value=1
  Switch : fl_lib/Electrical/Electrical Elements/Switch  R_closed=Ron Ohm  G_open=1e-8 1/Ohm  Threshold=7.5  i_specify=off  i_priority=None  i=0 A  i_nominal_specify=off  i_nominal_unit=A  i_nominal_value=1  v_specify=off  v_priority=None  v=0 V  v_nominal_specify=off  v_nominal_unit=V  v_nominal_value=1
  G : PMIOPort  Side=Left
  C : PMIOPort  Port=2  Side=Left
  E : PMIOPort  Port=3  Side=Right
  connections:
  Switch/RConn2 -- C/RConn1 -- Diode/RConn1
  Switch/RConn1 -- G/RConn1
  Switch/LConn1 -- E/RConn1 -- Diode/LConn1

== system two_parallel_full_model_simscape/zvs_modB/zvs_ctrl/vi ctrl/Iout Ctrl/iout_ctrl ==
  i_tilde : Inport
  1/Ti : Gain  Gain=kp_i_zvs  ParamDataTypeStr=double  OutDataTypeStr=double  SaturateOnIntegerOverflow=on
  Saturation2 : Saturate  UpperLimit=1  LowerLimit=0  OutDataTypeStr=double
  Sum1 : Sum  Inputs=+++  SaturateOnIntegerOverflow=on
  Sum4 : Sum  Inputs=-+  SaturateOnIntegerOverflow=on
  Unit Delay4 : UnitDelay  SampleTime=ts_zvs  HasFrameUpgradeWarning=on
  kp2 : Gain  Gain=ki_i_zvs*ts_zvs  ParamDataTypeStr=double  OutDataTypeStr=double  SaturateOnIntegerOverflow=on
  ctrli_out : Outport
  wires:
  Unit Delay4/1 -> Sum1/3
  Sum4/1 -> Unit Delay4/1
  1/Ti/1 -> Sum4/1, Sum1/1
  kp2/1 -> Sum1/2
  Saturation2/1 -> ctrli_out/1, Sum4/2
  Sum1/1 -> Saturation2/1
  i_tilde/1 -> 1/Ti/1, kp2/1

== system two_parallel_full_model_simscape/zvs_modB/zvs_ctrl/vi ctrl/Vout Ctrl/vout_ctrl ==
  ixi_tilde : Inport
  1/Ti : Gain  Gain=kp_v_zvs  ParamDataTypeStr=double  OutDataTypeStr=double  SaturateOnIntegerOverflow=on
  Saturation2 : Saturate  UpperLimit=1  LowerLimit=0  OutDataTypeStr=double
  Sum1 : Sum  Inputs=+++  SaturateOnIntegerOverflow=on
  Sum4 : Sum  Inputs=-+  SaturateOnIntegerOverflow=on
  Unit Delay4 : UnitDelay  SampleTime=ts_zvs  HasFrameUpgradeWarning=on
  kp2 : Gain  Gain=ki_v_zvs*ts_zvs  ParamDataTypeStr=double  OutDataTypeStr=double  SaturateOnIntegerOverflow=on
  ctrlv_out : Outport
  wires:
  Saturation2/1 -> Sum4/2, ctrlv_out/1
  Unit Delay4/1 -> Sum1/3
  Sum1/1 -> Saturation2/1
  1/Ti/1 -> Sum4/1, Sum1/1
  Sum4/1 -> Unit Delay4/1
  kp2/1 -> Sum1/2
  ixi_tilde/1 -> 1/Ti/1, kp2/1

== matlab function two_parallel_full_model_simscape/inverter_modA/single phase inverter control/pwm/PWM generator 2/MATLAB Function ==
  data: t input; y output; phase input; period input
function y = trgo(t,phase,period)
x = sin(2*pi/period*t - phase - pi/2);
y = asin(x);

== matlab function two_parallel_full_model_simscape/inverter_modB/single phase inverter control/flt_dq_d_i1 ==
  data: input input; y output
function y  = flt_dq_d(input)

FLTD2Q_B1 = 0.000966531084866133;
FLTD2Q_B2 = 0.000946498544476605;
FLTD2Q_A1 = -1.93814485260962;
FLTD2Q_A2 = 0.939101367424292;

    persistent x1 x2 y1 y2

    if isempty(x1)
        x1=0;
        x2=0;
        y1=0;
        y2=0;
    end


    o = x1 * FLTD2Q_B1 + x2 * FLTD2Q_B2 - y1 * FLTD2Q_A1 - y2 * FLTD2Q_A2;
    x2 = x1;
    x1 = input;
    y2 = y1;
    y1 = o;
	y = o;
end

== matlab function two_parallel_full_model_simscape/grid/grid_emulator/grid_source/phase_gen/bounder1 ==
  data: u input; y output
function y = bounder(u)
    
    y = -pi + mod(u+3*pi,2*pi);
end

== matlab function two_parallel_full_model_simscape/grid/grid_emulator/grid_source/voltage_grid/alphabeta2abc ==
  data: alpha input; a output; beta input; b output; c output
function [a,b,c] = alphabeta2abc(alpha,beta)

    a  =  alpha;
    b  =  -0.5*alpha + sqrt(3)/2*beta;
    c  =  -0.5*alpha - sqrt(3)/2*beta;
end

== matlab function two_parallel_full_model_simscape/grid/grid_emulator/grid_source/voltage_grid/xieta2alphabeta_neg ==
  data: xi input; alpha output; eta input; gamma input; beta output
function [alpha,beta] = xieta2alphabeta_neg(xi,eta,gamma)

    alpha  =  xi*cos(gamma) + eta*sin(gamma);
    beta = -xi*sin(gamma) + eta*cos(gamma);

end

== matlab function two_parallel_full_model_simscape/grid/grid_emulator/grid_source/voltage_grid/xieta2alphabeta_pos ==
  data: xi input; alpha output; eta input; gamma input; beta output
function [alpha,beta] = xieta2alphabeta_pos(xi,eta,gamma)

    alpha  =  xi*cos(gamma) - eta*sin(gamma);
    beta = xi*sin(gamma) + eta*cos(gamma);

end

== matlab function two_parallel_full_model_simscape/inverter_modA/phase_gen/bounder1 ==
  data: u input; y output
function y = bounder(u)
    
    y = -pi + mod(u+3*pi,2*pi);
end

== matlab function two_parallel_full_model_simscape/inverter_modA/single phase inverter control/flt_dq_d_i ==
  data: input input; y output
function y  = flt_dq_d(input)

FLTD2Q_B1 = 0.000966531084866133;
FLTD2Q_B2 = 0.000946498544476605;
FLTD2Q_A1 = -1.93814485260962;
FLTD2Q_A2 = 0.939101367424292;

    persistent x1 x2 y1 y2

    if isempty(x1)
        x1=0;
        x2=0;
        y1=0;
        y2=0;
    end


    o = x1 * FLTD2Q_B1 + x2 * FLTD2Q_B2 - y1 * FLTD2Q_A1 - y2 * FLTD2Q_A2;
    x2 = x1;
    x1 = input;
    y2 = y1;
    y1 = o;
	y = o;
end

== matlab function two_parallel_full_model_simscape/inverter_modA/single phase inverter control/flt_dq_d_u ==
  data: input input; y output
function y  = flt_dq_d(input)

FLTD2Q_B1 = 0.000966531084866133;
FLTD2Q_B2 = 0.000946498544476605;
FLTD2Q_A1 = -1.93814485260962;
FLTD2Q_A2 = 0.939101367424292;

    persistent x1 x2 y1 y2

    if isempty(x1)
        x1=0;
        x2=0;
        y1=0;
        y2=0;
    end


    o = x1 * FLTD2Q_B1 + x2 * FLTD2Q_B2 - y1 * FLTD2Q_A1 - y2 * FLTD2Q_A2;
    x2 = x1;
    x1 = input;
    y2 = y1;
    y1 = o;
	y = o;
end

== matlab function two_parallel_full_model_simscape/inverter_modB/single phase inverter control/flt_dq_d_i ==
  data: input input; y output
function y  = flt_dq_d(input)

FLTD2Q_B1 = 0.000966531084866133;
FLTD2Q_B2 = 0.000946498544476605;
FLTD2Q_A1 = -1.93814485260962;
FLTD2Q_A2 = 0.939101367424292;

    persistent x1 x2 y1 y2

    if isempty(x1)
        x1=0;
        x2=0;
        y1=0;
        y2=0;
    end


    o = x1 * FLTD2Q_B1 + x2 * FLTD2Q_B2 - y1 * FLTD2Q_A1 - y2 * FLTD2Q_A2;
    x2 = x1;
    x1 = input;
    y2 = y1;
    y1 = o;
	y = o;
end

== matlab function two_parallel_full_model_simscape/inverter_modB/phase_gen/bounder1 ==
  data: u input; y output
function y = bounder(u)
    
    y = -pi + mod(u+3*pi,2*pi);
end

== matlab function two_parallel_full_model_simscape/inverter_modB/single phase inverter control/pwm/PWM generator 1/MATLAB Function ==
  data: t input; y output; phase input; period input
function y = trgo(t,phase,period)
x = sin(2*pi/period*t - phase - pi/2);
y = asin(x);

== matlab function two_parallel_full_model_simscape/inverter_modB/single phase inverter control/pwm/PWM generator 2/MATLAB Function ==
  data: t input; y output; phase input; period input
function y = trgo(t,phase,period)
x = sin(2*pi/period*t - phase - pi/2);
y = asin(x);

== matlab function two_parallel_full_model_simscape/inverter_modA/single phase inverter control/pwm/PWM generator 1/MATLAB Function ==
  data: t input; y output; phase input; period input
function y = trgo(t,phase,period)
x = sin(2*pi/period*t - phase - pi/2);
y = asin(x);
